simulink model "Extended_17_level_inverter"  (R2020a)
settings: Solver=VariableStepAuto  StartTime=0.0  StopTime=1  RelTol=1e-3  EnableMultiTasking=on
libraries: powerlib x26
settings Model: Creator=shahin  LastModifiedBy=shahinSabour
settings DataIOCC: ReturnWorkspaceOutputs=off
settings OptimizationCC: LifeSpan=inf
settings DebuggingCC: SFUnexpectedBacktrackingDiag=warning  SFNoUnconditionalDefaultTransitionDiag=warning  ArithmeticOperatorsInVariantConditions=warning
settings SFSimCC: SimUseLocalCustomCode=off  CustomCodeUndefinedFunction=UseInterfaceOnly
settings RTWCC: RTWUseLocalCustomCode=off
settings CodeAppCC: StateflowObjectComments=on
settings GRTTargetCC: TargetLangStandard=C89/C90 (ANSI)
settings ConfigComp: CovMetricSettings=dw  CovHtmlReporting=on  CovSaveCumulativeToWorkspaceVar=on  CovSaveSingleToWorkspaceVar=on  CovExternalEMLEnable=off
settings SimscapeCC: SimscapeNormalizeSystem=off

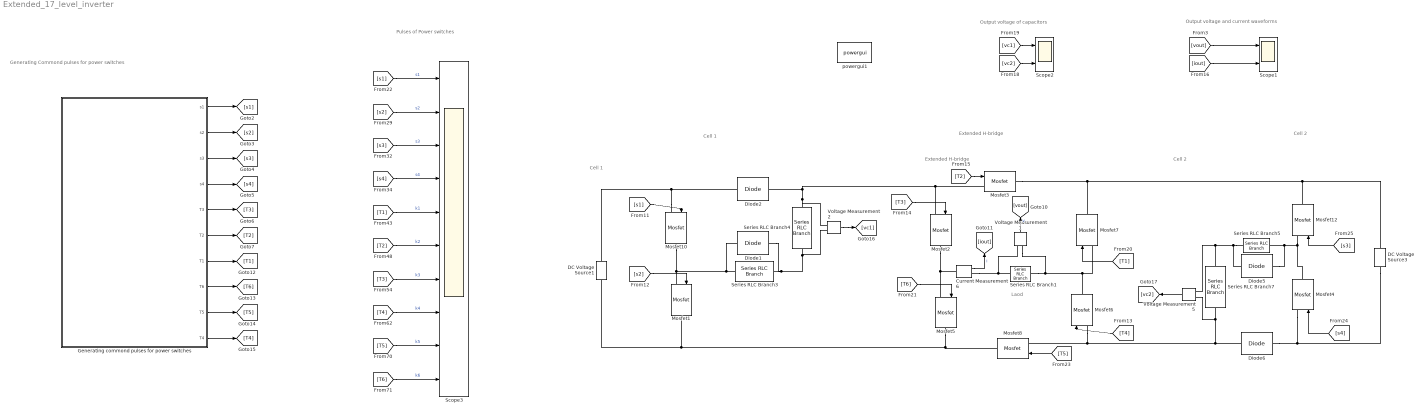
== system Extended_17_level_inverter ==
  note: Laod
  note: Extended H-bridge
  note: Cell 2
  note: Cell 1
  note: Output voltage of capacitors
  note: Output voltage and current waveforms
  note: Cell 1
  note: Cell 2
  note: Extended H-bridge
  note: Pulses of Power switches
  note: Generating Commond pulses for power switches
  Current Measurement6 : powerlib/Measurements/Current Measurement  PhasorSimulation=off  OutputType=Complex  PSBequivalent=0
  DC Voltage Source1 : powerlib/Electrical Sources/DC Voltage Source  Amplitude=50  Measurements=None
  DC Voltage Source3 : powerlib/Electrical Sources/DC Voltage Source  Amplitude=150  Measurements=None
  Diode{1..2,5..6} (4 alike) : powerlib/Power Electronics/Diode  Ron=0.001  Lon=0  Vf=0.8  IC=0  UseSnubber=off  Rs=500  Cs=250e-9  Measurements=off
  Generating commond pulses for power switches : Subsystem
  Mosfet{1..8,10,12} (10 alike) : powerlib/Power Electronics/Mosfet  Ron=0.1  Lon=0  Rd=0.01  Vfd=0  IC=0  Rs=1e5  Cs=inf  Measurements=off
  Scope1 : Scope  NumInputPorts=2
  Scope2 : Scope  NumInputPorts=2
  Scope3 : Scope  NumInputPorts=10
  Series RLC Branch1 : powerlib/Elements/Series RLC Branch  LConnTagsString=__new0  RConnTagsString=__new0  BranchType=RL  Resistance=40  Inductance=150e-3  SetiL0=off  InitialCurrent=0  Capacitance=1e-6  Setx0=off  InitialVoltage=0  Measurements=None
  Series RLC Branch3 : powerlib/Elements/Series RLC Branch  LConnTagsString=__new0  RConnTagsString=__new0  BranchType=L  Resistance=.1  Inductance=1000e-6  SetiL0=off  InitialCurrent=0  Capacitance=1e-6  Setx0=off  InitialVoltage=0  Measurements=None
  Series RLC Branch4 : powerlib/Elements/Series RLC Branch  LConnTagsString=__new0  RConnTagsString=__new0  BranchType=C  Resistance=1  Inductance=1e-6  SetiL0=off  InitialCurrent=0  Capacitance=2000e-6  Setx0=off  InitialVoltage=0  Measurements=None
  Series RLC Branch5 : powerlib/Elements/Series RLC Branch  LConnTagsString=__new0  RConnTagsString=__new0  BranchType=L  Resistance=.1  Inductance=1000e-6  SetiL0=off  InitialCurrent=0  Capacitance=1e-6  Setx0=off  InitialVoltage=0  Measurements=None
  Series RLC Branch7 : powerlib/Elements/Series RLC Branch  LConnTagsString=__new0  RConnTagsString=__new0  BranchType=C  Resistance=1  Inductance=1e-6  SetiL0=off  InitialCurrent=0  Capacitance=2000e-6  Setx0=off  InitialVoltage=0  Measurements=None
  Voltage Measurement1 : powerlib/Measurements/Voltage Measurement  PhasorSimulation=off  OutputType=Complex  PSBequivalent=0
  Voltage Measurement2 : powerlib/Measurements/Voltage Measurement  PhasorSimulation=off  OutputType=Complex  PSBequivalent=0
  Voltage Measurement5 : powerlib/Measurements/Voltage Measurement  PhasorSimulation=off  OutputType=Complex  PSBequivalent=0
  powergui1 : powerlib/powergui  Priority=1  SimulationMode=Discrete  SampleTime=50e-6  frequency=60  Iterations=50  frequencyindice=0  Pbase=100e6  ErrMax=1e-4  UnitsV=kV  UnitsW=MW  buscounter=0  FunctionMessages=off  echomessages=off  EnableUseOfTLC=off  CurrentSourceSwitches=off  DisableSnubberDevices=off  DisableRonSwitches=off  DisableVfSwitches=off  DisplayEquations=off  AutomaticDiscreteSolvers=off  SolverType=Tustin/Backward Euler (TBE)  Interpol=off  ExternalGateDelay=off  methode=off  Ts=10  x0status=blocks  SPID=off  SwTol=0  HookPort=off  NonlinearTolerance=1e-4  nMaxIteration=100  ContinueOnMaxIteration=off  RestoreLinks=warning  ResistiveCurrentMeasurement=off  Frange=[0:2:500]  Ylog=off  Xlog=on  ShowGrid=off  save=off  variable=ZData  structure=ibab  ZoomFFT=off  StartTime=0.6  cycles=2  DisplayStyle=1  fundamental=50  FreqAxis=on  MaxFrequency=1000  frequencyindicesteady=1  RmsSteady=1  display=off
  wires:
  Generating commond pulses for power switches/1(s1) -> [s1]
  Generating commond pulses for power switches/2(s2) -> [s2]
  Generating commond pulses for power switches/3(s3) -> [s3]
  Generating commond pulses for power switches/4(s4) -> [s4]
  Generating commond pulses for power switches/5(T3) -> [T3]
  Generating commond pulses for power switches/6(T2) -> [T2]
  Generating commond pulses for power switches/7(T1) -> [T1]
  Generating commond pulses for power switches/8(T6) -> [T6]
  Generating commond pulses for power switches/9(T5) -> [T5]
  Generating commond pulses for power switches/10(T4) -> [T4]
  [s1] -> Scope3/1  "s1"
  [s2] -> Scope3/2  "s2"
  [s3] -> Scope3/3  "s3"
  [s4] -> Scope3/4  "s4"
  [T1] -> Scope3/5  "k1"
  [T2] -> Scope3/6  "k2"
  [T3] -> Scope3/7  "k3"
  [T4] -> Scope3/8  "k4"
  [T5] -> Scope3/9  "k5"
  [T6] -> Scope3/10  "k6"
  [iout] -> Scope1/2
  [vout] -> Scope1/1
  [vc1] -> Scope2/1
  [vc2] -> Scope2/2
  [s2] -> Mosfet1/1
  Voltage Measurement2/1 -> [vc1]
  [s3] -> Mosfet12/1
  [s1] -> Mosfet10/1
  Current Measurement6/1 -> [iout]  "i"
  [T4] -> Mosfet6/1
  Voltage Measurement1/1 -> [vout]  "v"
  [T1] -> Mosfet7/1
  [T2] -> Mosfet3/1
  [T3] -> Mosfet2/1
  [T6] -> Mosfet5/1
  [T5] -> Mosfet8/1
  Voltage Measurement5/1 -> [vc2]
  [s4] -> Mosfet4/1
  connections:
  Mosfet10/LConn1 -- Diode2/LConn1 -- DC Voltage Source1/RConn1
  Series RLC Branch3/LConn1 -- Diode1/LConn1 -- Mosfet10/RConn1 -- Mosfet1/LConn1
  Mosfet5/RConn1 -- Mosfet8/RConn1 -- DC Voltage Source1/LConn1 -- Mosfet1/RConn1
  Diode1/RConn1 -- Voltage Measurement2/LConn2 -- Series RLC Branch4/RConn1 -- Series RLC Branch3/RConn1
  DC Voltage Source3/RConn1 -- Mosfet4/LConn1 -- Diode6/LConn1
  Series RLC Branch5/RConn1 -- Voltage Measurement5/LConn2 -- Series RLC Branch7/LConn1 -- Diode5/RConn1
  Mosfet12/LConn1 -- Mosfet4/RConn1 -- Diode5/LConn1 -- Series RLC Branch5/LConn1
  Current Measurement6/RConn1 -- Voltage Measurement1/LConn1 -- Series RLC Branch1/LConn1
  Mosfet12/RConn1 -- Mosfet7/RConn1 -- Mosfet3/RConn1 -- DC Voltage Source3/LConn1
  Series RLC Branch1/RConn1 -- Voltage Measurement1/LConn2 -- Mosfet6/RConn1 -- Mosfet7/LConn1
  Mosfet2/RConn1 -- Current Measurement6/LConn1 -- Mosfet5/LConn1
  Voltage Measurement2/LConn1 -- Series RLC Branch4/LConn1 -- Diode2/RConn1 -- Mosfet2/LConn1 -- Mosfet3/LConn1
  Diode6/RConn1 -- Series RLC Branch7/RConn1 -- Voltage Measurement5/LConn1 -- Mosfet6/LConn1 -- Mosfet8/LConn1

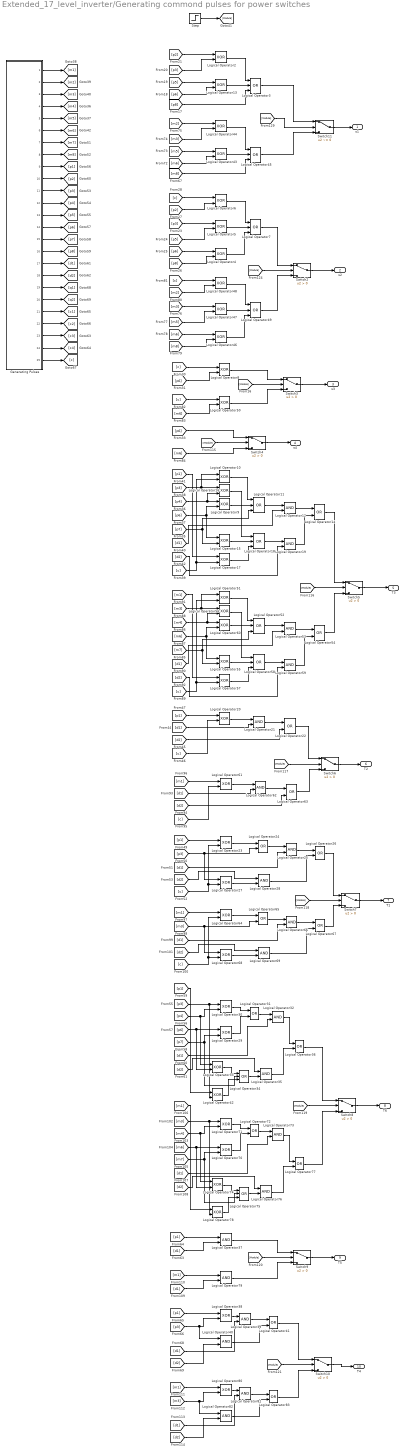
== system Extended_17_level_inverter/Generating commond pulses for power switches ==
  Generating Pulses : Subsystem
  Logical Operator{2,4..6,8..10,13,15..17,20,23,27,29..30,33,38,42..44,46..48,50..51,55..57,60..61,64,68,70..71,74,78,80} (38 alike) : Logic  Operator=XOR  AllPortsSameDT=off  OutDataTypeStr=boolean
  Logical Operator{3,7,11,18,34,45,49,52,58,75} (10 alike) : Logic  Operator=OR  Inputs=3  AllPortsSameDT=off  OutDataTypeStr=boolean
  Logical Operator{12,19,21,25,28,32,35,37,39..40,53,59,62,66,69,73,76,79,81..82} (20 alike) : Logic  AllPortsSameDT=off  OutDataTypeStr=boolean
  Logical Operator{14,22,24,26,31,36,41,54,63,65,67,72,77,83} (14 alike) : Logic  Operator=OR  AllPortsSameDT=off  OutDataTypeStr=boolean
  Step : Step  Before=1  After=0  SampleTime=0
  Switch{2..10} (9 alike) : Switch  Criteria=u2 > Threshold
  Switch11 : Switch  Criteria=u2 ~= 0
  s1 : Outport
  s2 : Outport  Port=2
  s3 : Outport  Port=3
  s4 : Outport  Port=4
  T3 : Outport  Port=5
  T2 : Outport  Port=6
  T1 : Outport  Port=7
  T6 : Outport  Port=8
  T5 : Outport  Port=9
  T4 : Outport  Port=10
  wires:
  [p5] -> Logical Operator5/2
  [p2] -> Logical Operator6/2
  [c] -> Logical Operator6/1
  Logical Operator6/1 -> Logical Operator7/1
  [p5] -> Logical Operator13/1
  [p8] -> Logical Operator4/2
  [p6] -> Logical Operator13/2
  [p3] -> Logical Operator2/2
  [p2] -> Logical Operator2/1
  Logical Operator2/1 -> Logical Operator3/1
  [p8] -> Logical Operator3/3
  [p6] -> Logical Operator4/1
  Logical Operator13/1 -> Logical Operator3/2
  [p3] -> Logical Operator5/1
  Logical Operator11/1 -> Logical Operator12/1
  Logical Operator9/1 -> Logical Operator11/2
  Logical Operator12/1 -> Logical Operator14/1
  [c] -> Logical Operator8/1
  [d1] -> Logical Operator12/2
  [p7] -> Logical Operator15/2, Logical Operator11/3
  [c] -> Logical Operator20/2
  Logical Operator4/1 -> Logical Operator7/3
  Logical Operator10/1 -> Logical Operator11/1
  Logical Operator20/1 -> Logical Operator21/1
  [d1] -> Logical Operator21/2
  [p1] -> Logical Operator17/1
  [p3] -> Logical Operator16/1, Logical Operator10/1
  Logical Operator15/1 -> Logical Operator18/2
  [p6] -> Logical Operator8/2
  [c] -> Logical Operator17/2, Logical Operator10/2
  [p4] -> Logical Operator9/1, Logical Operator16/2
  Logical Operator5/1 -> Logical Operator7/2
  Logical Operator16/1 -> Logical Operator18/1
  Logical Operator17/1 -> Logical Operator18/3
  [p1] -> Logical Operator20/1
  [p6] -> Logical Operator15/1, Logical Operator9/2
  Logical Operator18/1 -> Logical Operator19/1
  [d2] -> Logical Operator19/2
  Logical Operator19/1 -> Logical Operator14/2
  Logical Operator21/1 -> Logical Operator22/1
  [d2] -> Logical Operator22/2
  [p3] -> Logical Operator42/2, Logical Operator30/1
  Logical Operator23/1 -> Logical Operator24/1
  [p7] -> Logical Operator34/2, Logical Operator29/2
  Logical Operator38/1 -> Logical Operator39/1
  Logical Operator32/1 -> Logical Operator36/1
  [p4] -> Logical Operator33/1, Logical Operator30/2
  Logical Operator28/1 -> Logical Operator26/2
  [p1] -> Logical Operator38/1
  [c] -> Logical Operator27/2, Logical Operator23/2
  Logical Operator29/1 -> Logical Operator31/2
  [p3] -> Logical Operator40/1, Logical Operator38/2
  Logical Operator25/1 -> Logical Operator26/1
  [d1] -> Logical Operator25/2
  [p1] -> Logical Operator37/1
  [d2] -> Logical Operator35/1
  [d1] -> Logical Operator39/2
  Logical Operator39/1 -> Logical Operator41/1
  [p6] -> Logical Operator33/2, Logical Operator29/1
  Logical Operator30/1 -> Logical Operator31/1
  [d2] -> Logical Operator28/1
  [d1] -> Logical Operator37/2
  Logical Operator34/1 -> Logical Operator35/2
  [p1] -> Logical Operator23/1
  Logical Operator27/1 -> Logical Operator28/2
  [p3] -> Logical Operator24/2, Logical Operator27/1
  Logical Operator24/1 -> Logical Operator25/1
  Logical Operator31/1 -> Logical Operator32/1
  [d1] -> Logical Operator32/2
  Logical Operator35/1 -> Logical Operator36/2
  [d2] -> Logical Operator40/2
  Logical Operator40/1 -> Logical Operator41/2
  [p1] -> Logical Operator42/1
  Logical Operator33/1 -> Logical Operator34/1
  Logical Operator42/1 -> Logical Operator34/3
  [m2] -> Logical Operator44/1
  [m3] -> Logical Operator44/2
  Logical Operator44/1 -> Logical Operator45/1
  Logical Operator43/1 -> Logical Operator45/2
  [m8] -> Logical Operator45/3
  Step/1 -> [Module]
  [m5] -> Logical Operator43/1
  [m6] -> Logical Operator43/2
  [d2] -> Logical Operator59/2
  Logical Operator59/1 -> Logical Operator54/2
  Logical Operator55/1 -> Logical Operator58/2
  [m1] -> Logical Operator61/1
  [c] -> Logical Operator51/2, Logical Operator57/2
  [m7] -> Logical Operator52/3, Logical Operator55/2
  [c] -> Logical Operator61/2
  Logical Operator56/1 -> Logical Operator58/1
  Logical Operator61/1 -> Logical Operator62/1
  Logical Operator53/1 -> Logical Operator54/1
  [d1] -> Logical Operator62/2
  [m8] -> Logical Operator46/2
  [c] -> Logical Operator48/1
  Logical Operator57/1 -> Logical Operator58/3
  [m6] -> Logical Operator50/2
  [m6] -> Logical Operator60/2, Logical Operator55/1
  [m5] -> Logical Operator47/2
  [m2] -> Logical Operator48/2
  [m4] -> Logical Operator56/2, Logical Operator60/1
  [m3] -> Logical Operator51/1, Logical Operator56/1
  Logical Operator48/1 -> Logical Operator49/1
  Logical Operator51/1 -> Logical Operator52/1
  [m6] -> Logical Operator46/1
  Logical Operator46/1 -> Logical Operator49/3
  [d1] -> Logical Operator53/2
  [m1] -> Logical Operator57/1
  Logical Operator47/1 -> Logical Operator49/2
  [m3] -> Logical Operator47/1
  [c] -> Logical Operator50/1
  Logical Operator60/1 -> Logical Operator52/2
  Logical Operator52/1 -> Logical Operator53/1
  Logical Operator58/1 -> Logical Operator59/1
  [m3] -> Logical Operator82/1, Logical Operator80/2
  Logical Operator71/1 -> Logical Operator72/1
  [d1] -> Logical Operator66/2
  [m7] -> Logical Operator70/2, Logical Operator75/2
  [m3] -> Logical Operator71/1, Logical Operator78/2
  [m4] -> Logical Operator71/2, Logical Operator74/1
  Logical Operator62/1 -> Logical Operator63/1
  Logical Operator70/1 -> Logical Operator72/2
  [m3] -> Logical Operator68/1, Logical Operator65/2
  Logical Operator76/1 -> Logical Operator77/2
  [m1] -> Logical Operator78/1
  Logical Operator69/1 -> Logical Operator67/2
  Logical Operator78/1 -> Logical Operator75/3
  [d2] -> Logical Operator63/2
  [d2] -> Logical Operator69/1
  [d1] -> Logical Operator73/2
  [m1] -> Logical Operator80/1
  Logical Operator80/1 -> Logical Operator81/1
  Logical Operator74/1 -> Logical Operator75/1
  Logical Operator73/1 -> Logical Operator77/1
  Logical Operator64/1 -> Logical Operator65/1
  Logical Operator65/1 -> Logical Operator66/1
  Logical Operator68/1 -> Logical Operator69/2
  [c] -> Logical Operator64/2, Logical Operator68/2
  [m6] -> Logical Operator70/1, Logical Operator74/2
  [d2] -> Logical Operator76/1
  Logical Operator72/1 -> Logical Operator73/1
  Logical Operator66/1 -> Logical Operator67/1
  Logical Operator75/1 -> Logical Operator76/2
  [m1] -> Logical Operator64/1
  [d1] -> Logical Operator79/2
  [m1] -> Logical Operator79/1
  [Module] -> Switch2/2
  Switch4/1 -> s4/1
  [Module] -> Switch8/2
  Switch6/1 -> T2/1
  Logical Operator81/1 -> Logical Operator83/1
  Switch5/1 -> T3/1
  Logical Operator63/1 -> Switch6/3
  [Module] -> Switch10/2
  Logical Operator8/1 -> Switch3/1
  [m6] -> Switch4/3
  Logical Operator82/1 -> Logical Operator83/2
  [Module] -> Switch9/2
  Switch10/1 -> T4/1
  Logical Operator14/1 -> Switch5/1
  [Module] -> Switch4/2
  Logical Operator22/1 -> Switch6/1
  Switch8/1 -> T6/1
  Logical Operator26/1 -> Switch7/1
  [d2] -> Logical Operator82/2
  [Module] -> Switch5/2
  [Module] -> Switch3/2
  Switch2/1 -> s2/1
  [Module] -> Switch6/2
  [d1] -> Logical Operator81/2
  Switch7/1 -> T1/1
  Switch9/1 -> T5/1
  Logical Operator7/1 -> Switch2/1
  [Module] -> Switch7/2
  Logical Operator49/1 -> Switch2/3
  Logical Operator50/1 -> Switch3/3
  [p6] -> Switch4/1
  Logical Operator54/1 -> Switch5/3
  Logical Operator83/1 -> Switch10/3
  Logical Operator37/1 -> Switch9/1
  Switch3/1 -> s3/1
  Logical Operator79/1 -> Switch9/3
  Logical Operator67/1 -> Switch7/3
  Logical Operator41/1 -> Switch10/1
  Logical Operator3/1 -> Switch11/1
  Switch11/1 -> s1/1
  Logical Operator77/1 -> Switch8/3
  [Module] -> Switch11/2
  Logical Operator45/1 -> Switch11/3
  Logical Operator36/1 -> Switch8/1
  Generating Pulses/1(1) -> [m1]
  Generating Pulses/2(2) -> [m2]
  Generating Pulses/3(3) -> [m3]
  Generating Pulses/4(4) -> [m4]
  Generating Pulses/5(5) -> [m5]
  Generating Pulses/6(6) -> [m6]
  Generating Pulses/7(7) -> [m7]
  Generating Pulses/8(8) -> [m8]
  Generating Pulses/9(9) -> [p1]
  Generating Pulses/10(10) -> [p2]
  Generating Pulses/11(11) -> [p3]
  Generating Pulses/12(12) -> [p4]
  Generating Pulses/13(13) -> [p5]
  Generating Pulses/14(14) -> [p6]
  Generating Pulses/15(15) -> [p7]
  Generating Pulses/16(16) -> [p8]
  Generating Pulses/17(17) -> [d1]
  Generating Pulses/18(18) -> [d2]
  Generating Pulses/19(19) -> [q1]
  Generating Pulses/20(20) -> [q2]
  Generating Pulses/21(21) -> [c1]
  Generating Pulses/22(22) -> [c2]
  Generating Pulses/23(23) -> [c3]
  Generating Pulses/24(24) -> [c4]
  Generating Pulses/25(25) -> [c]

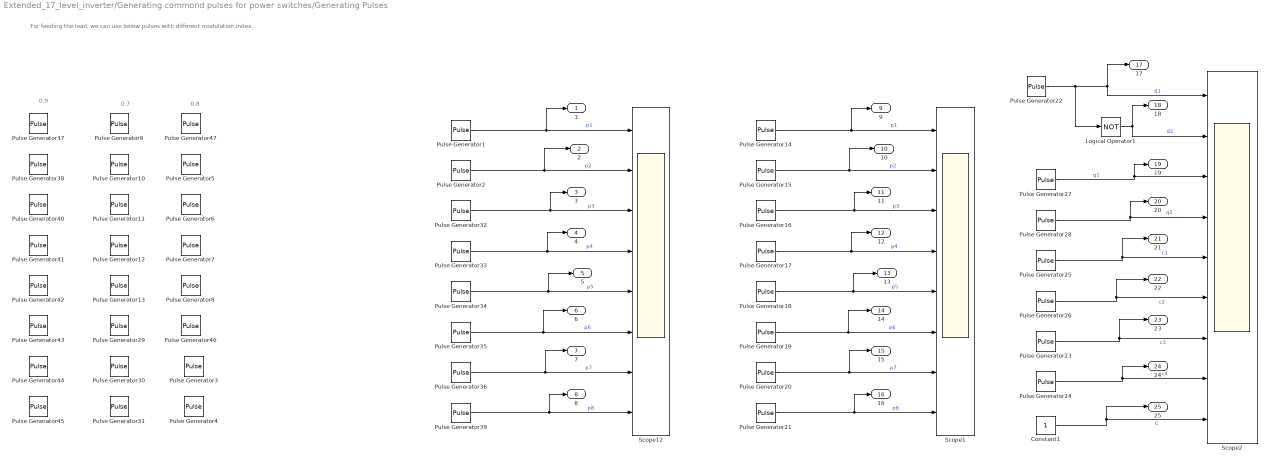
== system Extended_17_level_inverter/Generating commond pulses for power switches/Generating Pulses ==
  note: For feeding the load, we can use below pulses
      | with different modulation index.
  note: 0.8
  note: 0.7
  note: 0.9
  Constant1 : Constant
  Logical Operator1 : Logic  Operator=NOT  AllPortsSameDT=off  OutDataTypeStr=boolean
  Pulse Generator1 : DiscretePulseGenerator  PulseType=Time based  Period=.01  PulseWidth=95%  PhaseDelay=.0002  VectorParams1D=off
  Pulse Generator10 : DiscretePulseGenerator  PulseType=Time based  Period=.01  PulseWidth=82%  PhaseDelay=.00085  VectorParams1D=off
  Pulse Generator11 : DiscretePulseGenerator  PulseType=Time based  Period=.01  PulseWidth=70%  PhaseDelay=.0014  VectorParams1D=off
  Pulse Generator12 : DiscretePulseGenerator  PulseType=Time based  Period=.01  PulseWidth=57%  PhaseDelay=.0021  VectorParams1D=off
  Pulse Generator13 : DiscretePulseGenerator  PulseType=Time based  Period=.01  PulseWidth=40%  PhaseDelay=.0029  VectorParams1D=off
  Pulse Generator14 : DiscretePulseGenerator  PulseType=Time based  Period=.01  PulseWidth=96%  PhaseDelay=.000197  VectorParams1D=off
  Pulse Generator15 : DiscretePulseGenerator  PulseType=Time based  Period=.01  PulseWidth=88%  PhaseDelay=.00059  VectorParams1D=off
  Pulse Generator16 : DiscretePulseGenerator  PulseType=Time based  Period=.01  PulseWidth=79%  PhaseDelay=.001  VectorParams1D=off
  Pulse Generator17 : DiscretePulseGenerator  PulseType=Time based  Period=.01  PulseWidth=71%  PhaseDelay=.00143  VectorParams1D=off
  Pulse Generator18 : DiscretePulseGenerator  PulseType=Time based  Period=.01  PulseWidth=62%  PhaseDelay=.00187  VectorParams1D=off
  Pulse Generator19 : DiscretePulseGenerator  PulseType=Time based  Period=.01  PulseWidth=51%  PhaseDelay=.0024  VectorParams1D=off
  Pulse Generator2 : DiscretePulseGenerator  PulseType=Time based  Period=.01  PulseWidth=86%  PhaseDelay=.00066  VectorParams1D=off
  Pulse Generator20 : DiscretePulseGenerator  PulseType=Time based  Period=.01  PulseWidth=40%  PhaseDelay=.0029  VectorParams1D=off
  Pulse Generator21 : DiscretePulseGenerator  PulseType=Time based  Period=.01  PulseWidth=23%  PhaseDelay=.0038  VectorParams1D=off
  Pulse Generator22 : DiscretePulseGenerator  PulseType=Time based  Period=1/50  PulseWidth=50%  VectorParams1D=off
  Pulse Generator23 : DiscretePulseGenerator  PulseType=Time based  Period=1/50  PulseWidth=25%  PhaseDelay=.01  VectorParams1D=off
  Pulse Generator24 : DiscretePulseGenerator  PulseType=Time based  Period=1/50  PulseWidth=25%  PhaseDelay=.015  VectorParams1D=off
  Pulse Generator25 : DiscretePulseGenerator  PulseType=Time based  Period=1/50  PulseWidth=25%  VectorParams1D=off
  Pulse Generator26 : DiscretePulseGenerator  PulseType=Time based  Period=1/50  PulseWidth=25%  PhaseDelay=.005  VectorParams1D=off
  Pulse Generator27 : DiscretePulseGenerator  PulseType=Time based  Period=.01  PulseWidth=50%  VectorParams1D=off
  Pulse Generator28 : DiscretePulseGenerator  PulseType=Time based  Period=.01  PulseWidth=50%  PhaseDelay=.005  VectorParams1D=off
  Pulse Generator29 : DiscretePulseGenerator  PulseType=Time based  Period=.01  PulseWidth=12%  PhaseDelay=.0043  VectorParams1D=off
  Pulse Generator3 : DiscretePulseGenerator  PulseType=Time based  Period=.01  PulseWidth=0.000001  PhaseDelay=.0032  VectorParams1D=off
  Pulse Generator30 : DiscretePulseGenerator  PulseType=Time based  Period=.01  PulseWidth=0.0001  PhaseDelay=.0035  VectorParams1D=off
  Pulse Generator31 : DiscretePulseGenerator  PulseType=Time based  Period=.01  PulseWidth=0.0001  PhaseDelay=.0031  VectorParams1D=off
  Pulse Generator32 : DiscretePulseGenerator  PulseType=Time based  Period=.01  PulseWidth=77%  PhaseDelay=.0011  VectorParams1D=off
  Pulse Generator33 : DiscretePulseGenerator  PulseType=Time based  Period=.01  PulseWidth=68%  PhaseDelay=.0015  VectorParams1D=off
  Pulse Generator34 : DiscretePulseGenerator  PulseType=Time based  Period=.01  PulseWidth=57%  PhaseDelay=.0021  VectorParams1D=off
  Pulse Generator35 : DiscretePulseGenerator  PulseType=Time based  Period=.01  PulseWidth=45%  PhaseDelay=.0027  VectorParams1D=off
  Pulse Generator36 : DiscretePulseGenerator  PulseType=Time based  Period=.01  PulseWidth=28%  PhaseDelay=.0035  VectorParams1D=off
  Pulse Generator37 : DiscretePulseGenerator  PulseType=Time based  Period=.01  PulseWidth=95%  PhaseDelay=.0002  VectorParams1D=off
  Pulse Generator38 : DiscretePulseGenerator  PulseType=Time based  Period=.01  PulseWidth=86%  PhaseDelay=.00066  VectorParams1D=off
  Pulse Generator39 : DiscretePulseGenerator  PulseType=Time based  Period=.01  PulseWidth=0.0001  PhaseDelay=.0031  VectorParams1D=off
  Pulse Generator4 : DiscretePulseGenerator  PulseType=Time based  Period=.01  PulseWidth=0.000001  PhaseDelay=.0032  VectorParams1D=off
  Pulse Generator40 : DiscretePulseGenerator  PulseType=Time based  Period=.01  PulseWidth=77%  PhaseDelay=.0011  VectorParams1D=off
  Pulse Generator41 : DiscretePulseGenerator  PulseType=Time based  Period=.01  PulseWidth=68%  PhaseDelay=.0015  VectorParams1D=off
  Pulse Generator42 : DiscretePulseGenerator  PulseType=Time based  Period=.01  PulseWidth=57%  PhaseDelay=.0021  VectorParams1D=off
  Pulse Generator43 : DiscretePulseGenerator  PulseType=Time based  Period=.01  PulseWidth=45%  PhaseDelay=.0027  VectorParams1D=off
  Pulse Generator44 : DiscretePulseGenerator  PulseType=Time based  Period=.01  PulseWidth=28%  PhaseDelay=.0035  VectorParams1D=off
  Pulse Generator45 : DiscretePulseGenerator  PulseType=Time based  Period=.01  PulseWidth=0.0001  PhaseDelay=.0031  VectorParams1D=off
  Pulse Generator46 : DiscretePulseGenerator  PulseType=Time based  Period=.01  PulseWidth=34%  PhaseDelay=.0032  VectorParams1D=off
  Pulse Generator47 : DiscretePulseGenerator  PulseType=Time based  Period=.01  PulseWidth=95%  PhaseDelay=.0002  VectorParams1D=off
  Pulse Generator5 : DiscretePulseGenerator  PulseType=Time based  Period=.01  PulseWidth=85%  PhaseDelay=.00073  VectorParams1D=off
  Pulse Generator6 : DiscretePulseGenerator  PulseType=Time based  Period=.01  PulseWidth=74%  PhaseDelay=.0012  VectorParams1D=off
  Pulse Generator7 : DiscretePulseGenerator  PulseType=Time based  Period=.01  PulseWidth=63%  PhaseDelay=.0018  VectorParams1D=off
  Pulse Generator8 : DiscretePulseGenerator  PulseType=Time based  Period=.01  PulseWidth=50%  PhaseDelay=.0024  VectorParams1D=off
  Pulse Generator9 : DiscretePulseGenerator  PulseType=Time based  Period=.01  PulseWidth=94%  PhaseDelay=.00028  VectorParams1D=off
  Scope1 : Scope  NumInputPorts=8
  Scope12 : Scope  NumInputPorts=8
  Scope2 : Scope  NumInputPorts=9
  1 : Outport
  2 : Outport  Port=2
  3 : Outport  Port=3
  4 : Outport  Port=4
  5 : Outport  Port=5
  6 : Outport  Port=6
  7 : Outport  Port=7
  8 : Outport  Port=8
  9 : Outport  Port=9
  10 : Outport  Port=10
  11 : Outport  Port=11
  12 : Outport  Port=12
  13 : Outport  Port=13
  14 : Outport  Port=14
  15 : Outport  Port=15
  16 : Outport  Port=16
  17 : Outport  Port=17
  18 : Outport  Port=18
  19 : Outport  Port=19
  20 : Outport  Port=20
  21 : Outport  Port=21
  22 : Outport  Port=22
  23 : Outport  Port=23
  24 : Outport  Port=24
  25 : Outport  Port=25
  wires:
  Pulse Generator21/1 -> 16/1, Scope1/8  "p8"
  Pulse Generator2/1 -> 2/1, Scope12/2  "p2"
  Pulse Generator28/1 -> 20/1, Scope2/4  "q2"
  Pulse Generator26/1 -> 22/1, Scope2/6  "c2"
  Pulse Generator35/1 -> 6/1, Scope12/6  "p6"
  Pulse Generator20/1 -> 15/1, Scope1/7  "p7"
  Pulse Generator18/1 -> 13/1, Scope1/5  "p5"
  Pulse Generator1/1 -> 1/1, Scope12/1  "p1"
  Pulse Generator24/1 -> 24/1, Scope2/8  "c4"
  Pulse Generator22/1 -> 17/1, Scope2/1, Logical Operator1/1  "d1"
  Pulse Generator14/1 -> 9/1, Scope1/1  "p1"
  Pulse Generator34/1 -> 5/1, Scope12/5  "p5"
  Pulse Generator39/1 -> 8/1, Scope12/8  "p8"
  Pulse Generator27/1 -> 19/1, Scope2/3  "q1"
  Pulse Generator16/1 -> 11/1, Scope1/3  "p3"
  Pulse Generator36/1 -> 7/1, Scope12/7  "p7"
  Pulse Generator19/1 -> 14/1, Scope1/6  "p6"
  Constant1/1 -> 25/1, Scope2/9  "C"
  Pulse Generator17/1 -> 12/1, Scope1/4  "p4"
  Pulse Generator15/1 -> 10/1, Scope1/2  "p2"
  Pulse Generator25/1 -> 21/1, Scope2/5  "c1"
  Pulse Generator33/1 -> 4/1, Scope12/4  "p4"
  Logical Operator1/1 -> 18/1, Scope2/2  "d2"
  Pulse Generator23/1 -> 23/1, Scope2/7  "c3"
  Pulse Generator32/1 -> 3/1, Scope12/3  "p3"
